simulink model "Multiplication"  (R2024a)
settings: Solver=FixedStepDiscrete  StartTime=0.0  StopTime=0.2  FixedStep=Ts  RelTol=1e-3
StartFcn:
  | tic
StopFcn:
  | toc
values from neighbouring files (symbols this model uses):
  f = 50    [Multiinit.m]
  N = 5    [Multiinit.m]
  N2 = 2*N    (= 10)    [Multiinit.m]
  Ts = 2e-5    (= 2e-05)    [Multiinit.m]
  Xdcpnz_c = [0 0 0 0.676112454069 0.108637556 0.517272211534 -0.219489218604 -0.0466780460181 -0.00535926570279 -0.118991395138 -0.516218947359 0.0958685772847 ... (18 elements, 3x6)]    [Xdcpnz_c.mat]
  Ydcpnz_c = [0 0 0 0.3547 -0.5594 -0.803 0.1234 -0.1194 0.6299 -0.2311 0.0133 0.5451 ... (18 elements, 3x6)]    [Ydcpnz_c.mat]
  Ydcpnz_c2 = [0 0 0 0.576790935647 0.0786136210256 0.271851676895 -0.123704883485 0.599082227437 0.0697472802392 0.225557989324 0.265593743324 0.028658635911 ... (33 elements, 3x11)]    [Ydcpnz_c2.mat]
libraries: DQsym_Lib x5, spspowerguiLib x1
settings Model: SimulationMode=accelerator  Creator=The MathWorks, Inc.  LastModifiedBy=salsarayreh
settings SolverCC: AlgebraicLoopSolver=TrustRegion
settings DataIOCC: SaveFormat=StructureWithTime  SaveOutput=off  SaveState=on  DSMLogging=off  SaveTime=off  ReturnWorkspaceOutputs=off
settings OptimizationCC: ReuseModelBlockBuffer=off  ExpressionDepthLimit=2147483647  LifeSpan=inf
settings DebuggingCC: UnderspecifiedInitializationDetection=Classic  MergeDetectMultiDrivingBlocksExec=none  SolverPrmCheckMsg=warning  FcnCallInpInsideContextMsg=warning  UnconnectedInputMsg=warning  UnconnectedOutputMsg=warning  UnconnectedLineMsg=warning  AllowSymbolicDim=off  StateNameClashWarn=warning  SFUnexpectedBacktrackingDiag=warning  SFNoUnconditionalDefaultTransitionDiag=warning  SFExecutionAtInitializationDiag=none  ArithmeticOperatorsInVariantConditions=warning
settings HardwareCC: ProdBitPerPointer=32  ProdBitPerSizeT=32  ProdBitPerPtrDiffT=32  ProdLargestAtomicFloat=None  ProdIntDivRoundTo=Undefined  ProdEndianess=Unspecified  ProdWordSize=32  ProdHWDeviceType=32-bit Generic
settings ModelReferenceCC: EnableRefExpFcnMdlSchedulingChecks=on  PropagateSignalLabelsOutOfModel=off
settings SFSimCC: SimUseLocalCustomCode=off  CustomCodeUndefinedFunction=UseInterfaceOnly
settings RTWCC: RTWUseLocalCustomCode=off  GPUComputeCapability=3.5
settings CodeAppCC: StateflowObjectComments=on
settings GRTTargetCC: TargetLangStandard=C89/C90 (ANSI)  CombineOutputUpdateFcns=off  GRTInterface=on
settings ConfigComp: CovMetricSettings=dw  CovSaveCumulativeToWorkspaceVar=on  CovSaveSingleToWorkspaceVar=on  CovExternalEMLEnable=off
settings SimscapeCC: SimscapeNormalizeSystem=off

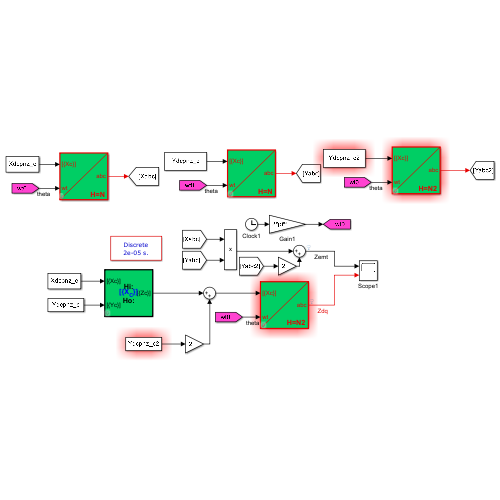
[thumbnail: Simulink's stored preview of the top-level diagram]
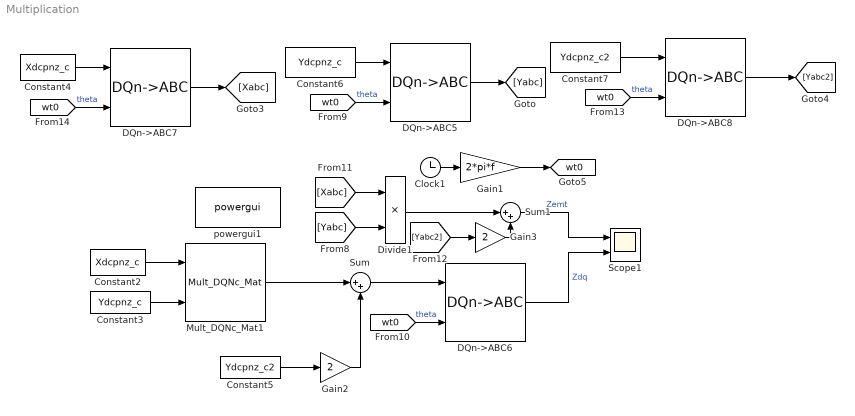
== system Multiplication ==
  Clock1 : Clock
  Constant2 : Constant  Value=Xdcpnz_c
  Constant3 : Constant  Value=Ydcpnz_c
  Constant4 : Constant  Value=Xdcpnz_c
  Constant5 : Constant  Value=Ydcpnz_c2
  Constant6 : Constant  Value=Ydcpnz_c
  Constant7 : Constant  Value=Ydcpnz_c2
  DQn->ABC5 : DQsym_Lib/DQn->ABC  N=N
      settings: SourceProductName=DQsym Library
  DQn->ABC6 : DQsym_Lib/DQn->ABC  N=N2
      settings: SourceProductName=DQsym Library
  DQn->ABC7 : DQsym_Lib/DQn->ABC  N=N
      settings: SourceProductName=DQsym Library
  DQn->ABC8 : DQsym_Lib/DQn->ABC  N=N2
      settings: SourceProductName=DQsym Library
  Divide1 : Product  Inputs=**
  Gain1 : Gain  Gain=2*pi*f
  Gain2 : Gain  Gain=2
  Gain3 : Gain  Gain=2
  Mult_DQNc_Mat1 : DQsym_Lib/Mult_DQNc_Mat  N=N  HrmDbl=on
      settings: SourceProductName=DQsym Library
  Scope1 : Scope  NumInputPorts=2
  Sum : Sum  Inputs=|++
  Sum1 : Sum  Inputs=|++
  powergui1 : spspowerguiLib/powergui  Priority=1  SimulationMode=Discrete  SampleTime=Ts  frequency=60  Iterations=50  frequencyindice=0  Pbase=100e6  ErrMax=1e-4  UnitsV=kV  UnitsW=MW  buscounter=0  FunctionMessages=off  echomessages=off  EnableUseOfTLC=off  CurrentSourceSwitches=off  DisableSnubberDevices=off  DisableRonSwitches=off  DisableVfSwitches=off  DisplayEquations=off  AutomaticDiscreteSolvers=off  SolverType=Tustin/Backward Euler (TBE)  Interpol=off  ExternalGateDelay=off  methode=off  Ts=10  x0status=blocks  SPID=off  SwTol=0  HookPort=off  NonlinearTolerance=1e-4  nMaxIteration=100  ContinueOnMaxIteration=off  RestoreLinks=warning  ResistiveCurrentMeasurement=off  Frange=[0:2:500]  Ylog=off  Xlog=on  ShowGrid=off  save=off  variable=ZData  structure=VIprim  ZoomFFT=on  StartTime=0.15  cycles=2  DisplayStyle=1  fundamental=50  FreqAxis=on  MaxFrequency=1000  frequencyindicesteady=1  RmsSteady=1  display=off
  tag scope: wt0=global
  wires:
  Constant7/1 -> DQn->ABC8/1
  [Xabc] -> Divide1/1
  Constant5/1 -> Gain2/1
  [Yabc2] -> Gain3/1
  Gain2/1 -> Sum/2
  Gain3/1 -> Sum1/2
  Constant2/1 -> Mult_DQNc_Mat1/1
  Constant3/1 -> Mult_DQNc_Mat1/2
  Mult_DQNc_Mat1/1 -> Sum/1
  Divide1/1 -> Sum1/1
  DQn->ABC5/1 -> [Yabc]
  DQn->ABC8/1 -> [Yabc2]
  [wt0] -> DQn->ABC5/2  "theta"
  Sum/1 -> DQn->ABC6/1
  Constant4/1 -> DQn->ABC7/1
  [wt0] -> DQn->ABC6/2  "theta"
  [wt0] -> DQn->ABC7/2  "theta"
  [wt0] -> DQn->ABC8/2  "theta"
  Constant6/1 -> DQn->ABC5/1
  [Yabc] -> Divide1/2
  Gain1/1 -> [wt0]
  DQn->ABC6/1 -> Scope1/2  "Zdq"
  Clock1/1 -> Gain1/1
  DQn->ABC7/1 -> [Xabc]
  Sum1/1 -> Scope1/1  "Zemt"
